simulink model "IEEexperiment_3"  (R2024a)
settings: Solver=VariableStepAuto  StartTime=0.0  StopTime=10.0  RelTol=1e-3
libraries: spsSeriesRLCBranchLib x15, spsDCVoltageSourceLib x4, spspowerguiLib x4, spsCurrentMeasurementLib x3, spsImpedanceMeasurementLib x1, spsVoltageMeasurementLib x1, sps_lib x1
settings Model: Creator=LENOVO  LastModifiedBy=LENOVO

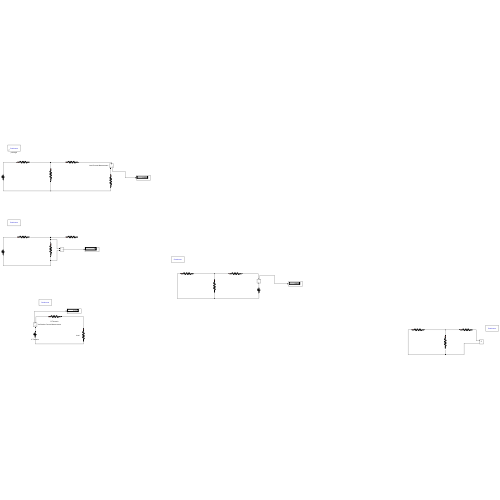
[thumbnail: Simulink's stored preview of the top-level diagram]
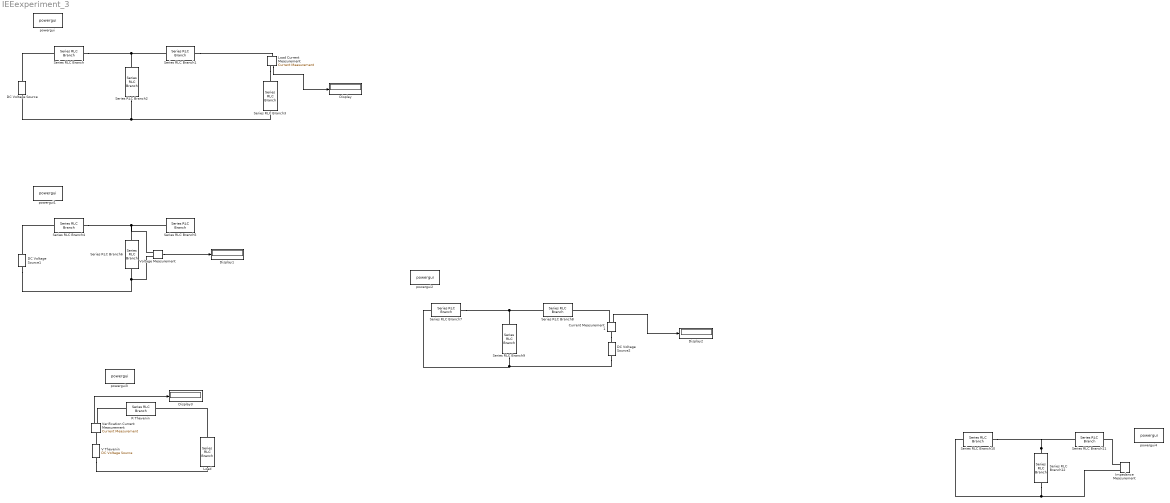
== system IEEexperiment_3 ==
  Current Measurement1 : spsCurrentMeasurementLib/Current Measurement  PhasorSimulation=off  OutputType=Complex  PSBequivalent=0
  DC Voltage Source : spsDCVoltageSourceLib/DC Voltage Source  Amplitude=30  Measurements=None
  DC Voltage Source1 : spsDCVoltageSourceLib/DC Voltage Source  Amplitude=30  Measurements=None
  DC Voltage Source2 : spsDCVoltageSourceLib/DC Voltage Source  Amplitude=30  Measurements=None
  Display{,1..3} (4 alike) : Display
  Impedance Measurement : spsImpedanceMeasurementLib/Impedance Measurement  LConnTagsString=+|-  Factor=1
      settings: LibrarySourceBlock=sps_lib/Sensors and Measurements/Impedance Measurement
  Load : spsSeriesRLCBranchLib/Series RLC Branch  LConnTagsString=__new0  RConnTagsString=__new0  BranchType=R  Resistance=10  Inductance=1e-3  SetiL0=off  InitialCurrent=0  Capacitance=1e-6  Setx0=off  InitialVoltage=0  Measurements=None
  "Load Current Measurement " : spsCurrentMeasurementLib/Current Measurement  PhasorSimulation=off  OutputType=Complex  PSBequivalent=0
  R Thevenin : spsSeriesRLCBranchLib/Series RLC Branch  LConnTagsString=__new0  RConnTagsString=__new0  BranchType=R  Resistance=63.331222292590  Inductance=1e-3  SetiL0=off  InitialCurrent=0  Capacitance=1e-6  Setx0=off  InitialVoltage=0  Measurements=None
  Series RLC Branch{,4,7,10} (4 alike) : spsSeriesRLCBranchLib/Series RLC Branch  LConnTagsString=__new0  RConnTagsString=__new0  BranchType=R  Resistance=20  Inductance=1e-3  SetiL0=off  InitialCurrent=0  Capacitance=1e-6  Setx0=off  InitialVoltage=0  Measurements=None
  Series RLC Branch{1,5,8,11} (4 alike) : spsSeriesRLCBranchLib/Series RLC Branch  LConnTagsString=__new0  RConnTagsString=__new0  BranchType=R  Resistance=50  Inductance=1e-3  SetiL0=off  InitialCurrent=0  Capacitance=1e-6  Setx0=off  InitialVoltage=0  Measurements=None
  Series RLC Branch{2,6,9,12} (4 alike) : spsSeriesRLCBranchLib/Series RLC Branch  LConnTagsString=__new0  RConnTagsString=__new0  BranchType=R  Resistance=40  Inductance=1e-3  SetiL0=off  InitialCurrent=0  Capacitance=1e-6  Setx0=off  InitialVoltage=0  Measurements=None
  Series RLC Branch3 : spsSeriesRLCBranchLib/Series RLC Branch  LConnTagsString=__new0  RConnTagsString=__new0  BranchType=R  Resistance=10  Inductance=1e-3  SetiL0=off  InitialCurrent=0  Capacitance=1e-6  Setx0=off  InitialVoltage=0  Measurements=None
  V Thevenin : spsDCVoltageSourceLib/DC Voltage Source  Amplitude=20  Measurements=None
  Verification Current Measurement : spsCurrentMeasurementLib/Current Measurement  PhasorSimulation=off  OutputType=Complex  PSBequivalent=0
  Voltage Measurement : spsVoltageMeasurementLib/Voltage Measurement  PhasorSimulation=off  OutputType=Complex  PSBequivalent=0
  powergui : sps_lib/powergui  Priority=1  SimulationMode=Continuous  SampleTime=50e-6  frequency=60  Iterations=50  frequencyindice=0  Pbase=100e6  ErrMax=1e-4  UnitsV=kV  UnitsW=MW  buscounter=0  FunctionMessages=off  echomessages=off  EnableUseOfTLC=off  CurrentSourceSwitches=off  DisableSnubberDevices=off  DisableRonSwitches=off  DisableVfSwitches=off  DisplayEquations=off  AutomaticDiscreteSolvers=off  SolverType=Tustin/Backward Euler (TBE)  Interpol=off  ExternalGateDelay=off  methode=off  Ts=100  x0status=blocks  SPID=on  SwTol=0  HookPort=off  NonlinearTolerance=1e-4  nMaxIteration=100  ContinueOnMaxIteration=off  RestoreLinks=warning  ResistiveCurrentMeasurement=off  Frange=[0:2:500]  Ylog=off  Xlog=on  ShowGrid=off  save=off  variable=ZData  structure=0  ZoomFFT=off  StartTime=0.0  cycles=1  DisplayStyle=1  fundamental=60  FreqAxis=off  MaxFrequency=1000  frequencyindicesteady=1  RmsSteady=1  display=off
  powergui{1..4} (4 alike) : spspowerguiLib/powergui  Priority=1  SimulationMode=Continuous  SampleTime=50e-6  frequency=60  Iterations=50  frequencyindice=0  Pbase=100e6  ErrMax=1e-4  UnitsV=kV  UnitsW=MW  buscounter=0  FunctionMessages=off  echomessages=off  EnableUseOfTLC=off  CurrentSourceSwitches=off  DisableSnubberDevices=off  DisableRonSwitches=off  DisableVfSwitches=off  DisplayEquations=off  AutomaticDiscreteSolvers=off  SolverType=Tustin/Backward Euler (TBE)  Interpol=off  ExternalGateDelay=off  methode=off  Ts=100  x0status=blocks  SPID=on  SwTol=0  HookPort=off  NonlinearTolerance=1e-4  nMaxIteration=100  ContinueOnMaxIteration=off  RestoreLinks=warning  ResistiveCurrentMeasurement=off  Frange=[0:2:500]  Ylog=off  Xlog=on  ShowGrid=off  save=off  variable=ZData  structure=0  ZoomFFT=off  StartTime=0.0  cycles=1  DisplayStyle=1  fundamental=60  FreqAxis=off  MaxFrequency=1000  frequencyindicesteady=1  RmsSteady=1  display=off
  wires:
  Voltage Measurement/1 -> Display1/1
  Current Measurement1/1 -> Display2/1
  "Load Current Measurement "/1 -> Display/1
  Verification Current Measurement/1 -> Display3/1
  connections:
  DC Voltage Source/RConn1 -- Series RLC Branch/LConn1
  Series RLC Branch/RConn1 -- Series RLC Branch1/LConn1 -- Series RLC Branch2/LConn1
  DC Voltage Source/LConn1 -- Series RLC Branch2/RConn1 -- Series RLC Branch3/RConn1
  Series RLC Branch1/RConn1 -- "Load Current Measurement "/LConn1
  "Load Current Measurement "/RConn1 -- Series RLC Branch3/LConn1
  Series RLC Branch4/RConn1 -- Voltage Measurement/LConn1 -- Series RLC Branch6/LConn1 -- Series RLC Branch5/LConn1
  DC Voltage Source1/LConn1 -- Voltage Measurement/LConn2 -- Series RLC Branch6/RConn1
  DC Voltage Source1/RConn1 -- Series RLC Branch4/LConn1
  Series RLC Branch7/RConn1 -- Series RLC Branch8/LConn1 -- Series RLC Branch9/LConn1
  Series RLC Branch9/RConn1 -- DC Voltage Source2/LConn1 -- Series RLC Branch7/LConn1
  Current Measurement1/LConn1 -- DC Voltage Source2/RConn1
  Current Measurement1/RConn1 -- Series RLC Branch8/RConn1
  V Thevenin/LConn1 -- Load/RConn1
  Load/LConn1 -- R Thevenin/RConn1
  V Thevenin/RConn1 -- Verification Current Measurement/LConn1
  Verification Current Measurement/RConn1 -- R Thevenin/LConn1
  Series RLC Branch12/RConn1 -- Series RLC Branch10/LConn1 -- Impedance Measurement/LConn2
  Series RLC Branch12/LConn1 -- Series RLC Branch10/RConn1 -- Series RLC Branch11/LConn1
  Impedance Measurement/LConn1 -- Series RLC Branch11/RConn1
